simulink model "MotorCtrl_V1"  (R2018a)
settings: configuration reference "Config_Ctrl" (kept outside this file)
PreLoadFcn:
  | MotorCtrl_V1_PreLoad
undefined symbols (not defined in the file): HevMotorGearRatio_K, HevMotorMaxTrq_K2, HevMotorMaxTrq_K2x
libraries: simulink x2
settings Model: Creator=IAEC nishito  LastModifiedBy=E00026
settings ConfigSetRef: SourceLocation=Base Workspace

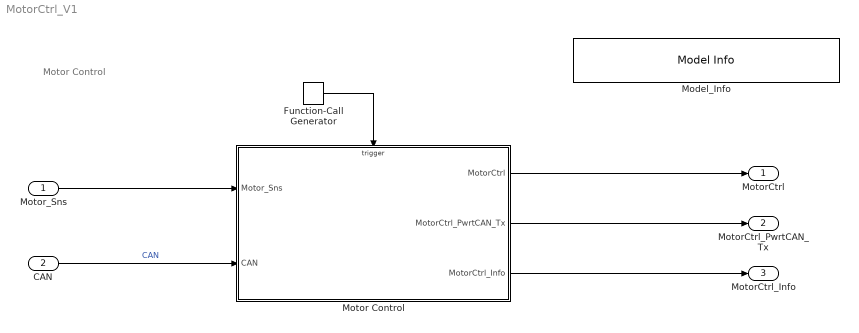
== system MotorCtrl_V1 ==
  note: Motor Control
  Motor_Sns : Inport  OutDataTypeStr=Bus:Motor_sensor_Bus
      settings: AttributesFormatString=%<OutDataTypeStr>
  CAN : Inport  Port=2  OutDataTypeStr=Bus: CAN_Bus
      settings: AttributesFormatString=<%<OutDataTypeStr>>
  Function-Call Generator : simulink/Ports & Subsystems/Function-Call Generator  sample_time=0.01  numberOfIterations=1
      settings: AttributesFormatString=<sample_time=%<sample_time>>
  Model_Info : simulink/Model-Wide Utilities/Model Info  Frame=on  DisplayStringWithTags=|  HorizontalTextAlignment=Left  LeftAlignmentValue=0.02
      | Version  %<ModelVersion>
      | LastModifided by %<LastModifiedBy>  Date %<LastModificationDate>
      | Description  %<Description>
  Motor Control : Subsystem
  MotorCtrl : Outport  OutDataTypeStr=Bus: MotorCtrl_Bus
      settings: AttributesFormatString=<%<OutDataTypeStr>>
  MotorCtrl_PwrtCAN_Tx : Outport  Port=2  OutDataTypeStr=Bus: MotorCtrl_PwtrCAN_Tx_Bus
      settings: AttributesFormatString=<%<OutDataTypeStr>>
  MotorCtrl_Info : Outport  Port=3  OutDataTypeStr=Bus: MotorCtrl_Info_Bus
      settings: AttributesFormatString=<%<OutDataTypeStr>>
  wires:
  CAN/1 -> Motor Control/2(CAN)  "CAN"
  Motor_Sns/1 -> Motor Control/1(Motor_Sns)
  Function-Call Generator/1 -> Motor Control/Trigger
  Motor Control/2(MotorCtrl_PwrtCAN_Tx) -> MotorCtrl_PwrtCAN_Tx/1
  Motor Control/1(MotorCtrl) -> MotorCtrl/1
  Motor Control/3(MotorCtrl_Info) -> MotorCtrl_Info/1

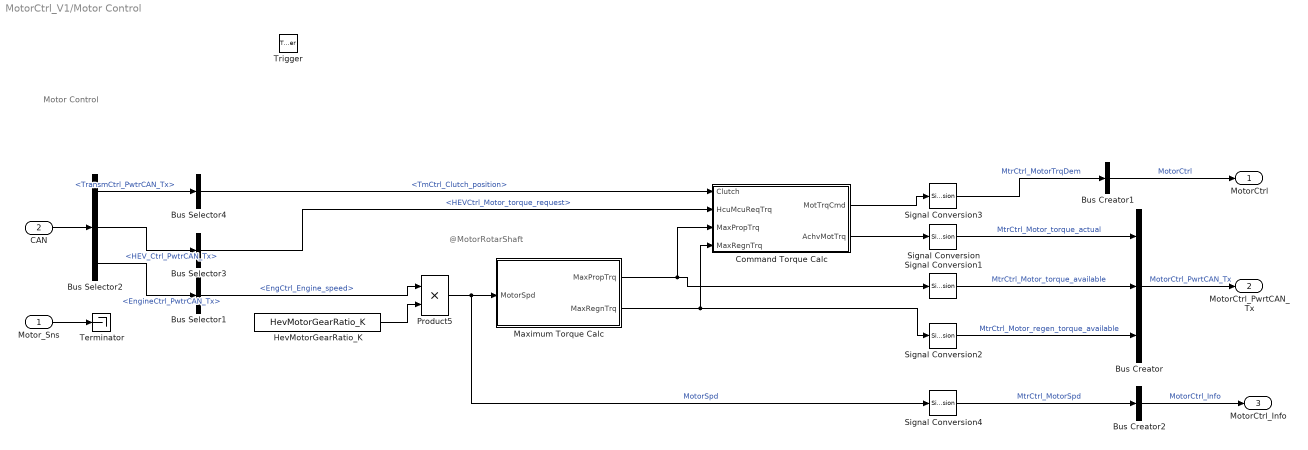
== system MotorCtrl_V1/Motor Control ==
  note: Motor Control
  note: ＠MotorRotarShaft
  Motor_Sns : Inport
  CAN : Inport  Port=2
  Trigger : TriggerPort  TriggerType=function-call  VariantControl=Variant  PortDimensions=1
  Bus Creator : BusCreator  Inputs=3  OutDataTypeStr=Bus: MotorCtrl_PwtrCAN_Tx_Bus
      settings: AttributesFormatString=%<OutDataTypeStr>
  Bus Creator1 : BusCreator  Inputs=1  OutDataTypeStr=Bus: MotorCtrl_Bus
      settings: AttributesFormatString=%<OutDataTypeStr>
  Bus Creator2 : BusCreator  Inputs=1  OutDataTypeStr=Bus: MotorCtrl_Info_Bus
      settings: AttributesFormatString=%<OutDataTypeStr>
  Bus Selector1 : BusSelector  OutputSignals=EngCtrl_Engine_speed
  Bus Selector2 : BusSelector  OutputSignals=PwtrCAN.TransmCtrl_PwtrCAN_Tx,PwtrCAN.HEV_Ctrl_PwtrCAN_Tx,PwtrCAN.EngineCtrl_PwtrCAN_Tx
  Bus Selector3 : BusSelector  OutputSignals=HEVCtrl_Motor_torque_request
  Bus Selector4 : BusSelector  OutputSignals=TmCtrl_Clutch_position
  Command Torque Calc : Subsystem
  "HevMotorGearRatio_K " : Constant  Value=HevMotorGearRatio_K
  Maximum Torque Calc : Subsystem
  Product5 : Product  RndMeth=Zero
  Signal Conversion{,1..4} (5 alike) : SignalConversion  OverrideOpt=off
  Terminator : Terminator
  MotorCtrl : Outport
  MotorCtrl_PwrtCAN_Tx : Outport  Port=2
  MotorCtrl_Info : Outport  Port=3
  wires:
  CAN/1 -> Bus Selector2/1
  Motor_Sns/1 -> Terminator/1
  Bus Creator/1 -> MotorCtrl_PwrtCAN_Tx/1  "MotorCtrl_PwrtCAN_Tx"
  Bus Creator1/1 -> MotorCtrl/1  "MotorCtrl"
  Bus Creator2/1 -> MotorCtrl_Info/1  "MotorCtrl_Info"
  Bus Selector2/2 -> Bus Selector3/1  "<HEV_Ctrl_PwtrCAN_Tx>"
  Command Torque Calc/2(AchvMotTrq) -> Signal Conversion/1
  Signal Conversion/1 -> Bus Creator/1  "MtrCtrl_Motor_torque_actual"
  Command Torque Calc/1(MotTrqCmd) -> Signal Conversion3/1
  Signal Conversion1/1 -> Bus Creator/2  "MtrCtrl_Motor_torque_available"
  Signal Conversion2/1 -> Bus Creator/3  "MtrCtrl_Motor_regen_torque_available"
  Signal Conversion3/1 -> Bus Creator1/1  "MtrCtrl_MotorTrqDem"
  Product5/1 -> Signal Conversion4/1, Maximum Torque Calc/1(MotorSpd)  "MotorSpd"
  Maximum Torque Calc/2(MaxRegnTrq) -> Command Torque Calc/4(MaxRegnTrq), Signal Conversion2/1
  Bus Selector4/1 -> Command Torque Calc/1(Clutch)  "<TmCtrl_Clutch_position>"
  "HevMotorGearRatio_K "/1 -> Product5/2
  Maximum Torque Calc/1(MaxPropTrq) -> Command Torque Calc/3(MaxPropTrq), Signal Conversion1/1
  Bus Selector1/1 -> Product5/1  "<EngCtrl_Engine_speed>"
  Bus Selector3/1 -> Command Torque Calc/2(HcuMcuReqTrq)  "<HEVCtrl_Motor_torque_request>"
  Bus Selector2/1 -> Bus Selector4/1  "<TransmCtrl_PwtrCAN_Tx>"
  Bus Selector2/3 -> Bus Selector1/1  "<EngineCtrl_PwtrCAN_Tx>"
  Signal Conversion4/1 -> Bus Creator2/1  "MtrCtrl_MotorSpd"

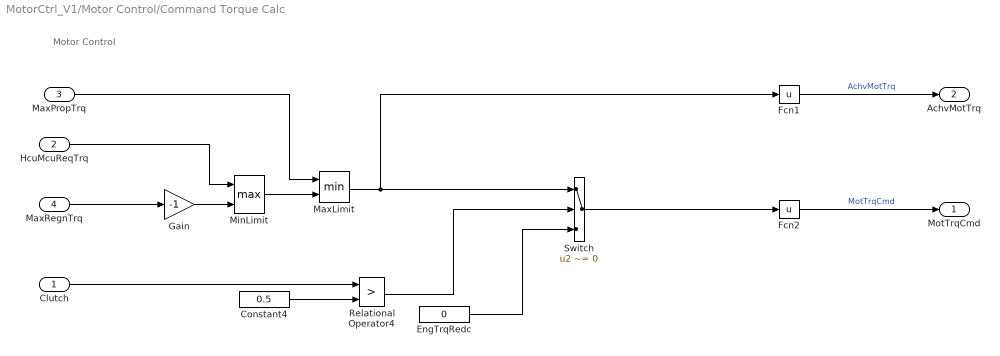
== system MotorCtrl_V1/Motor Control/Command Torque Calc ==
  note: Motor Control
  Clutch : Inport
  HcuMcuReqTrq : Inport  Port=2
  MaxPropTrq : Inport  Port=3
  MaxRegnTrq : Inport  Port=4
  Constant4 : Constant  Value=0.5
  EngTrqRedc : Constant  Value=0
  Fcn1 : Fcn  Expr=u
  Fcn2 : Fcn  Expr=u
  Gain : Gain  Gain=-1
  MaxLimit : MinMax  Inputs=2
  MinLimit : MinMax  Function=max  Inputs=2
  Relational Operator4 : RelationalOperator  Operator=>  OutDataTypeStr=boolean  RndMeth=Nearest
  Switch : Switch  Criteria=u2 ~= 0  Threshold=0.5  SaturateOnIntegerOverflow=on
      settings: AttributesFormatString=<%<Criteria>>
  MotTrqCmd : Outport
  AchvMotTrq : Outport  Port=2
  wires:
  Fcn1/1 -> AchvMotTrq/1  "AchvMotTrq"
  MaxRegnTrq/1 -> Gain/1
  Fcn2/1 -> MotTrqCmd/1  "MotTrqCmd"
  HcuMcuReqTrq/1 -> MinLimit/1
  MaxPropTrq/1 -> MaxLimit/1
  Gain/1 -> MinLimit/2
  MinLimit/1 -> MaxLimit/2
  MaxLimit/1 -> Switch/1, Fcn1/1
  Clutch/1 -> Relational Operator4/1
  Switch/1 -> Fcn2/1
  Constant4/1 -> Relational Operator4/2
  Relational Operator4/1 -> Switch/2
  EngTrqRedc/1 -> Switch/3

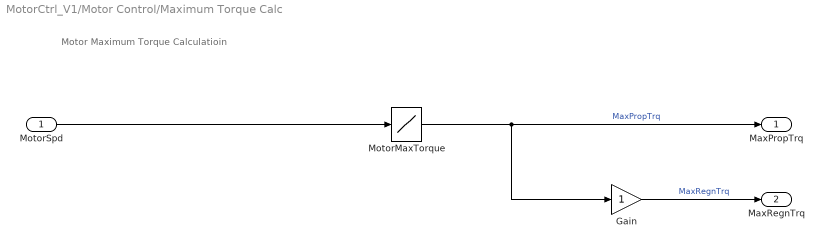
== system MotorCtrl_V1/Motor Control/Maximum Torque Calc ==
  note: Motor Maximum Torque Calculatioin
  MotorSpd : Inport
  Gain : Gain
  MotorMaxTorque : Lookup  InputValues=HevMotorMaxTrq_K2x  Table=HevMotorMaxTrq_K2  LookUpMeth=Interpolation-Use End Values  SaturateOnIntegerOverflow=on
      settings: AttributesFormatString=<input=%<InputValues>>\n<output=%<OutputValues>>
  MaxPropTrq : Outport
  MaxRegnTrq : Outport  Port=2
  wires:
  MotorMaxTorque/1 -> MaxPropTrq/1, Gain/1  "MaxPropTrq"
  MotorSpd/1 -> MotorMaxTorque/1
  Gain/1 -> MaxRegnTrq/1  "MaxRegnTrq"
